simulink library "Washout"  (Simulink 8.9)
settings: Solver=VariableStepAuto  StartTime=0.0  StopTime=10.0  RelTol=1e-3
settings Model: SuppressorTable=22 serialization::archive 11 0 6 0 0 0 0 0  Creator=hbolandhemmat  LastModifiedBy=hbolandhemmat

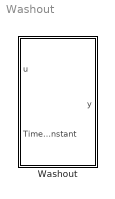
== system Washout ==
  Washout : Subsystem

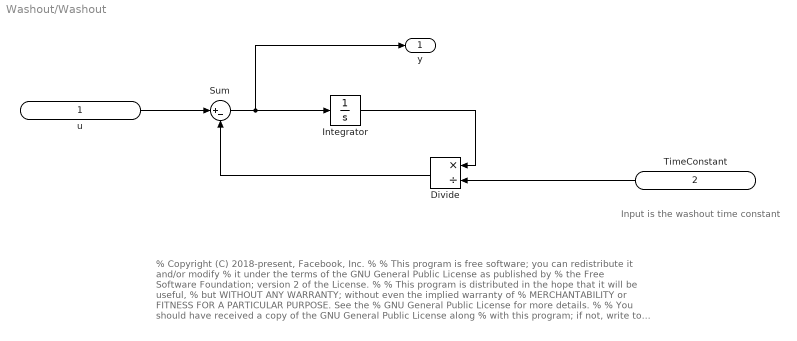
== system Washout/Washout ==
  note: Input is the washout time constant
  note: % Copyright (C) 2018-present, Facebook, Inc.
      | %
      | % This program is free software; you can redistribute it and/or modify
      | % it under the terms of the GNU General Public License as published by
      | % the Free Software Foundation; version 2 of the License.
      | %
      | % This program is distributed in the hope that it will be useful,
      | % but WITHOUT ANY WARRANTY; without even the implied warranty of
      | % MERCHANTABILITY or FITNESS FOR A PARTICULAR PURPOSE. See the
      | % GNU General Public License for more details.
      | %
      | % You should have received a copy of the GNU General Public License along
      | % with this program; if not, write to the Free Software Foundation, Inc.,
      | % 51 Franklin Street, Fifth Floor, Boston, MA 02110-1301 USA.
  u : Inport  OutDataTypeStr=double  PortDimensions=1  Interpolate=off
  TimeConstant : Inport  Port=2  OutDataTypeStr=double  PortDimensions=1  Interpolate=off
  Divide : Product  Inputs=*/
  Integrator : Integrator
  Sum : Sum  Inputs=|+-  InputSameDT=on  OutDataTypeStr=Inherit: Same as first input
  y : Outport  Description=Shall be used for all outputs except function outputs or nodes.
  wires:
  Integrator/1 -> Divide/1
  TimeConstant/1 -> Divide/2
  u/1 -> Sum/1
  Sum/1 -> Integrator/1, y/1
  Divide/1 -> Sum/2
